simulink model "Test_model"  (R2023a)
settings: Solver=FixedStepAuto  StartTime=0.0  StopTime=200  FixedStep=0.01  RelTol=1e-3
values from neighbouring files (symbols this model uses):
  shaft = struct("length", {})    [Shaft_data.m]
undefined symbols (not defined in the file or in its folder): moments
settings Model: Creator=User  LastModifiedBy=User

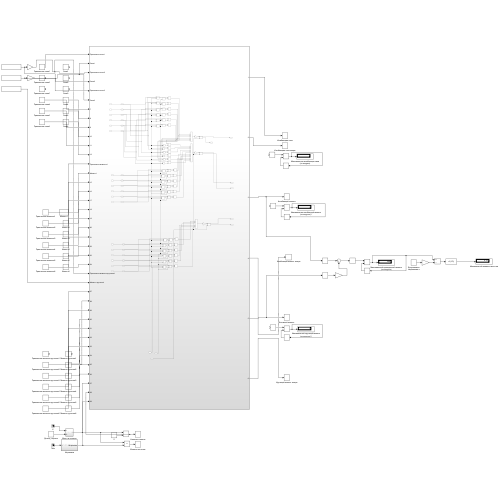
[thumbnail: Simulink's stored preview of the top-level diagram]
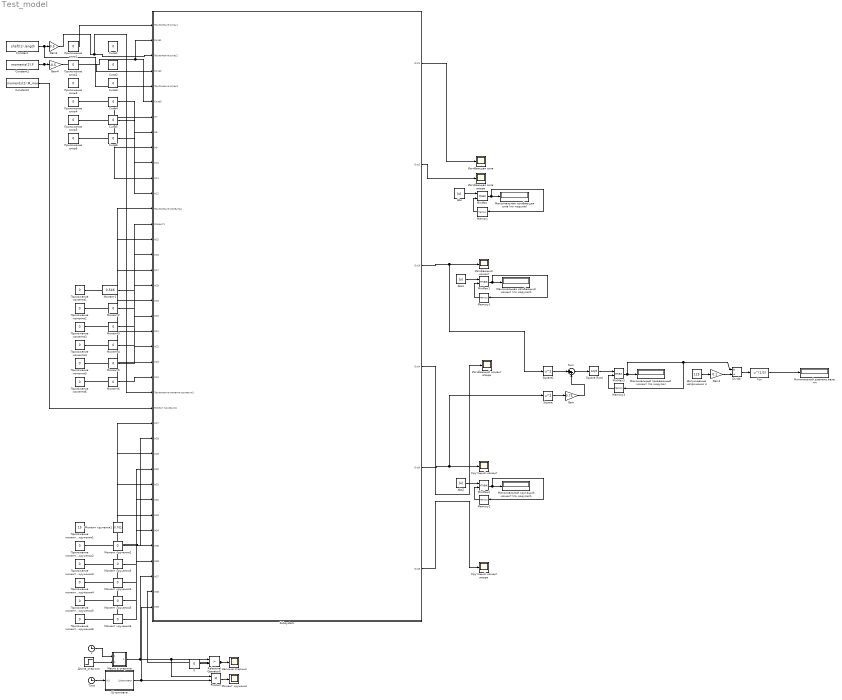
== system Test_model ==
  0 : Constant  Value=0
  Abs : Abs  SaturateOnIntegerOverflow=off
  Abs1 : Abs  SaturateOnIntegerOverflow=off
  Abs2 : Abs  SaturateOnIntegerOverflow=off
  Constant : Constant  Value=shaft(1).length
  Constant1 : Constant  Value=moments(2).F
  Constant2 : Constant  Value=moments(2).M_max
  Divide : Product  Inputs=*/
  Fcn : Fcn  Expr=u^(1/3)
  Gain : Gain  Gain=0.75
  Gain1 : Gain  Gain=0.1
  Gain3 : Gain  Gain=0.5
  Gain4 : Gain  Gain=-0.5
  Memory{,1..3} (4 alike) : Memory  InitialCondition=-10000
  MinMax{,1..3} (4 alike) : MinMax  Function=max  Inputs=2
  Product : Product
  Relational Operator6 : RelationalOperator  Operator=>  OutDataTypeStr=boolean  RndMeth=Simplest  InputSameDT=off
  Square : Math  Operator=square
  Square Root : Sqrt
  Square1 : Math  Operator=square
  Subsystem : Subsystem
  Sum : Sum  Inputs=|++
  Time : Clock
      settings: Decimation=15
  X : Clock
      settings: Decimation=15
  Длина_стержня : Step  Time=150  After=1000  SampleTime=0
  Допускаемые напряжения σ : Constant  Value=125
  Изгибающая сила : Scope
  Изгибающая сила эпюра : Scope
  Изгибающий момент : Scope
  Изгибающий момент эпюра : Scope
  Крутящий момент : Scope
  Крутящий момент эпюра : Scope
  Максимальная изгибающая сила (по модулю) : Display
  Максимальная изгибающий момент (по модулю)1 : Display
  Максимальный крутящий момент (по модулю)1 : Display
  Максимальный приведенный момент (по модулю) : Display
  Место в стержне : Subsystem
  "Минимальный диаметр вала, мм" : Display
  Момент кручения : Scope
  Момент кручения1 : Constant  Value=0.702
  Момент кручения{2..6} (5 alike) : Constant  Value=0
  Момент1 : Constant  Value=0.546
  Момент{2..6} (5 alike) : Constant  Value=0
  Наличие стержня : Scope
  Приложение момента кручения1 : Constant  Value=15
  Приложение момента кручения{2..6} (5 alike) : Constant  Value=0
  Приложение момента{1..6} (6 alike) : Constant  Value=0
  Приложение силы{1..6} (6 alike) : Constant  Value=0
  Сила{1..6} (6 alike) : Constant  Value=0
  Штриховка : Subsystem
  wires:
  Product/1 -> Момент кручения/1
  X/1 -> Место в стержне/1(In1)
  Длина_стержня/1 -> Место в стержне/2(In2)
  Time/1 -> Штриховка/1(In1)
  0/1 -> Relational Operator6/2
  MinMax/1 -> Максимальная изгибающая сила (по модулю)/1, Memory/1
  Memory/1 -> MinMax/2
  Штриховка/1(Штриховка) -> Product/2, Subsystem/39(In39)
  Relational Operator6/1 -> Наличие стержня/1, Subsystem/38(In38)
  Место в стержне/1(Out1) -> Relational Operator6/1, Product/1, Subsystem/37(In37)
  Subsystem/2(Out2) -> Изгибающая сила эпюра/1
  Приложение силы1/1 -> Subsystem/1(Приложение силы1)
  Приложение силы4/1 -> Subsystem/7(In7)
  Сила4/1 -> Subsystem/8(In8)
  Приложение силы5/1 -> Subsystem/9(In9)
  Сила5/1 -> Subsystem/10(In10)
  Приложение силы6/1 -> Subsystem/11(In11)
  Сила6/1 -> Subsystem/12(In12)
  Приложение момента1/1 -> Subsystem/13(Приложение момента1)
  Момент1/1 -> Subsystem/14(Момент1)
  Приложение момента2/1 -> Subsystem/15(In15)
  Момент2/1 -> Subsystem/16(In16)
  Приложение момента3/1 -> Subsystem/17(In17)
  Момент3/1 -> Subsystem/18(In18)
  Приложение момента4/1 -> Subsystem/19(In19)
  Момент4/1 -> Subsystem/20(In20)
  Приложение момента5/1 -> Subsystem/21(In21)
  Момент5/1 -> Subsystem/22(In22)
  Приложение момента6/1 -> Subsystem/23(In23)
  Момент6/1 -> Subsystem/24(In24)
  Приложение момента кручения2/1 -> Subsystem/27(In27)
  Момент кручения2/1 -> Subsystem/28(In28)
  Приложение момента кручения3/1 -> Subsystem/29(In29)
  Момент кручения3/1 -> Subsystem/30(In30)
  Приложение момента кручения4/1 -> Subsystem/31(In31)
  Момент кручения4/1 -> Subsystem/32(In32)
  Приложение момента кручения5/1 -> Subsystem/33(In33)
  Момент кручения5/1 -> Subsystem/34(In34)
  Приложение момента кручения6/1 -> Subsystem/35(In35)
  Момент кручения6/1 -> Subsystem/36(In36)
  Subsystem/1(Out1) -> Изгибающая сила/1
  Subsystem/3(Out3) -> Square1/1, Изгибающий момент/1
  Subsystem/4(Out4) -> Изгибающий момент эпюра/1
  Subsystem/5(Out5) -> Square/1, Крутящий момент/1
  Subsystem/6(Out6) -> Крутящий момент эпюра/1
  Abs/1 -> MinMax/1
  Abs1/1 -> MinMax1/1
  Memory1/1 -> MinMax1/2
  MinMax1/1 -> Максимальная изгибающий момент (по модулю)1/1, Memory1/1
  Abs2/1 -> MinMax2/1
  Memory2/1 -> MinMax2/2
  MinMax2/1 -> Максимальный крутящий момент (по модулю)1/1, Memory2/1
  Square/1 -> Gain/1
  Square1/1 -> Sum/1
  Gain/1 -> Sum/2
  Sum/1 -> Square Root/1
  Memory3/1 -> MinMax3/2
  MinMax3/1 -> Divide/1, Memory3/1, Максимальный приведенный момент (по модулю)/1
  Square Root/1 -> MinMax3/1
  Допускаемые напряжения σ/1 -> Gain1/1
  Gain1/1 -> Divide/2
  Divide/1 -> Fcn/1
  Fcn/1 -> "Минимальный диаметр вала, мм"/1
  Constant/1 -> Gain3/1, Subsystem/5(Приложение силы3)
  Gain3/1 -> Subsystem/25(Приложение момента кручения1), Subsystem/3(Приложение силы2)
  Constant1/1 -> Subsystem/4(Сила2), Gain4/1
  Gain4/1 -> Subsystem/6(Сила3), Subsystem/2(Сила1)
  Constant2/1 -> Subsystem/26(Момент кручения1)

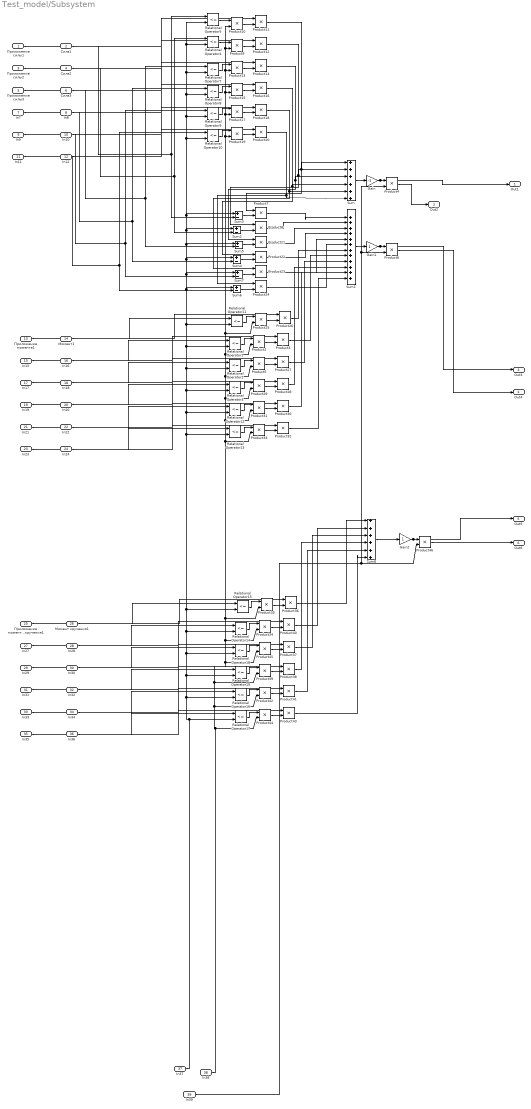
== system Test_model/Subsystem ==
  Приложение силы1 : Inport
  Сила1 : Inport  Port=2
  Приложение силы2 : Inport  Port=3
  Сила2 : Inport  Port=4
  Приложение силы3 : Inport  Port=5
  Сила3 : Inport  Port=6
  In7 : Inport  Port=7
  In8 : Inport  Port=8
  In9 : Inport  Port=9
  In10 : Inport  Port=10
  In11 : Inport  Port=11
  In12 : Inport  Port=12
  Приложение момента1 : Inport  Port=13
  Момент1 : Inport  Port=14
  In15 : Inport  Port=15
  In16 : Inport  Port=16
  In17 : Inport  Port=17
  In18 : Inport  Port=18
  In19 : Inport  Port=19
  In20 : Inport  Port=20
  In21 : Inport  Port=21
  In22 : Inport  Port=22
  In23 : Inport  Port=23
  In24 : Inport  Port=24
  Приложение момента кручения1 : Inport  Port=25
  Момент кручения1 : Inport  Port=26
  In27 : Inport  Port=27
  In28 : Inport  Port=28
  In29 : Inport  Port=29
  In30 : Inport  Port=30
  In31 : Inport  Port=31
  In32 : Inport  Port=32
  In33 : Inport  Port=33
  In34 : Inport  Port=34
  In35 : Inport  Port=35
  In36 : Inport  Port=36
  In37 : Inport  Port=37
  In38 : Inport  Port=38
  In39 : Inport  Port=39
  Gain : Gain  Gain=-1
  Gain1 : Gain
  Gain2 : Gain
  Product{2..46} (45 alike) : Product
  Relational Operator{1..5,7..19} (18 alike) : RelationalOperator  Operator=<=  OutDataTypeStr=boolean  RndMeth=Simplest  InputSameDT=off
  Sum : Sum  Inputs=|++++++
  Sum1 : Sum  Inputs=|++++++++++++
  Sum{2..7} (6 alike) : Sum  Inputs=|+-
  Sum8 : Sum  Inputs=|++++++
  Out1 : Outport
  Out2 : Outport  Port=2
  Out3 : Outport  Port=3
  Out4 : Outport  Port=4
  Out5 : Outport  Port=5
  Out6 : Outport  Port=6
  wires:
  In30/1 -> Product37/1
  Product20/1 -> Product24/1, Sum/6
  In38/1 -> Product44/2, Product42/2, Product39/2, Product45/2, Product35/2, Product33/2, Product31/2, Product29/2, Product5/2, Product2/2, Product25/2, Product19/2, Product17/2, Product15/2, Product13/2, Product10/2, Product9/2, Product34/2
  Sum8/1 -> Gain2/1
  Sum/1 -> Gain/1
  Product12/1 -> Product8/1, Sum/2
  Product18/1 -> Product23/1, Sum/5
  Relational Operator13/1 -> Product33/1
  In34/1 -> Product41/1
  Product24/1 -> Sum1/6
  Product39/1 -> Product38/2
  In37/1 -> Relational Operator17/2, Relational Operator19/2, Relational Operator18/2, Relational Operator14/2, Relational Operator15/2, Relational Operator12/2, Relational Operator1/2, Relational Operator11/2, Sum6/1, Sum7/1, Sum4/1, Sum5/1, Relational Operator10/2, Relational Operator9/2, Relational Operator7/2, Relational Operator5/2, Relational Operator4/2, Relational Operator8/2, Sum3/1, Sum2/1, Relational Operator2/2, Relational Operator3/2, Relational Operator13/2, Relational Operator16/2
  Product29/1 -> Product28/2
  Момент кручения1/1 -> Product36/1
  Relational Operator3/1 -> Product29/1
  In17/1 -> Relational Operator2/1
  Product14/1 -> Product21/1, Sum/3
  In11/1 -> Relational Operator10/1, Sum6/2
  Product11/1 -> Product7/1, Sum/1
  Relational Operator14/1 -> Product34/1
  In8/1 -> Product16/1
  Sum2/1 -> Product8/2
  Product16/1 -> Product22/1, Sum/4
  Product9/1 -> Product12/2
  Product33/1 -> Product32/2
  Relational Operator9/1 -> Product17/1
  Relational Operator10/1 -> Product19/1
  Сила3/1 -> Product14/1
  Product37/1 -> Sum8/3
  Product28/1 -> Sum1/10
  Product42/1 -> Product41/2
  Product4/1 -> Out2/1
  Product23/1 -> Sum1/5
  Product25/1 -> Product26/2
  In39/1 -> Product46/2, Product4/2, Product6/2
  Product34/1 -> Product40/2
  Relational Operator17/1 -> Product44/1
  Relational Operator16/1 -> Product42/1
  Relational Operator5/1 -> Product10/1
  Product36/1 -> Sum8/1
  Sum1/1 -> Gain1/1
  Relational Operator11/1 -> Product25/1
  Product8/1 -> Sum1/2
  Product32/1 -> Sum1/12
  Relational Operator7/1 -> Product13/1
  Sum3/1 -> Product7/2
  Product41/1 -> Sum8/5
  Product27/1 -> Sum1/9
  Product40/1 -> Sum8/2
  Product26/1 -> Sum1/7
  Product19/1 -> Product20/2
  Product30/1 -> Sum1/11
  Relational Operator15/1 -> Product35/1
  Relational Operator18/1 -> Product45/1
  Gain/1 -> Out1/1, Product4/1
  Приложение силы2/1 -> Sum2/2, Relational Operator4/1
  Product45/1 -> Product37/2
  Gain2/1 -> Out5/1, Product46/1
  Product7/1 -> Sum1/1
  In27/1 -> Relational Operator14/1
  Product17/1 -> Product18/2
  Приложение силы1/1 -> Sum3/2, Relational Operator5/1
  In9/1 -> Relational Operator9/1, Sum7/2
  Gain1/1 -> Out3/1, Product6/1
  Product13/1 -> Product14/2
  Приложение силы3/1 -> Relational Operator7/1, Sum5/2
  In33/1 -> Relational Operator16/1
  In22/1 -> Product30/1
  Relational Operator12/1 -> Product31/1
  In7/1 -> Relational Operator8/1, Sum4/2
  Product44/1 -> Product43/2
  Product3/1 -> Sum1/8
  Product38/1 -> Sum8/4
  Sum6/1 -> Product24/2
  Product21/1 -> Sum1/3
  Sum7/1 -> Product23/2
  Product31/1 -> Product30/2
  Sum5/1 -> Product21/2
  Sum4/1 -> Product22/2
  Relational Operator8/1 -> Product15/1
  Product15/1 -> Product16/2
  Relational Operator1/1 -> Product2/1
  In28/1 -> Product40/1
  Relational Operator2/1 -> Product5/1
  Relational Operator4/1 -> Product9/1
  Product2/1 -> Product3/2
  Product43/1 -> Sum8/6
  Product10/1 -> Product11/2
  Product5/1 -> Product27/2
  Product22/1 -> Sum1/4
  Relational Operator19/1 -> Product39/1
  Product35/1 -> Product36/2
  Product6/1 -> Out4/1
  Product46/1 -> Out6/1
  In29/1 -> Relational Operator18/1
  Момент1/1 -> Product26/1
  In35/1 -> Relational Operator17/1
  In19/1 -> Relational Operator3/1
  Приложение момента кручения1/1 -> Relational Operator15/1
  Сила2/1 -> Product12/1
  Приложение момента1/1 -> Relational Operator11/1
  In10/1 -> Product18/1
  In18/1 -> Product27/1
  In16/1 -> Product3/1
  In36/1 -> Product43/1
  In23/1 -> Relational Operator13/1
  In15/1 -> Relational Operator1/1
  In21/1 -> Relational Operator12/1
  In12/1 -> Product20/1
  In31/1 -> Relational Operator19/1
  In32/1 -> Product38/1
  In24/1 -> Product32/1
  In20/1 -> Product28/1
  Сила1/1 -> Product11/1

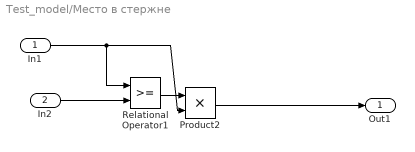
== system Test_model/Место в стержне ==
  In1 : Inport
  In2 : Inport  Port=2
  Product2 : Product
  Relational Operator1 : RelationalOperator  OutDataTypeStr=boolean  RndMeth=Simplest  InputSameDT=off
  Out1 : Outport
  wires:
  Relational Operator1/1 -> Product2/1
  Product2/1 -> Out1/1
  In2/1 -> Relational Operator1/2
  In1/1 -> Product2/2, Relational Operator1/1

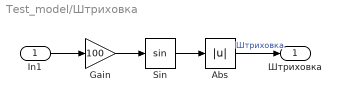
== system Test_model/Штриховка ==
  In1 : Inport
  Abs : Abs  SaturateOnIntegerOverflow=off
  Gain : Gain  Gain=100
  Sin : Trigonometry
  Штриховка : Outport
  wires:
  Sin/1 -> Abs/1
  In1/1 -> Gain/1
  Gain/1 -> Sin/1
  Abs/1 -> Штриховка/1  "Штриховка"
